simulink model "modelo_completo_2"  (R2023b)
settings: Solver=VariableStepAuto  StartTime=0.0  StopTime=300  MaxStep=5e-3  RelTol=1e-3
values from neighbouring files (symbols this model uses):
  P_p = 3    [constantes.m]
libraries: simulink x3
settings Model: Creator=Nahuel  LastModifiedBy=Nahuel

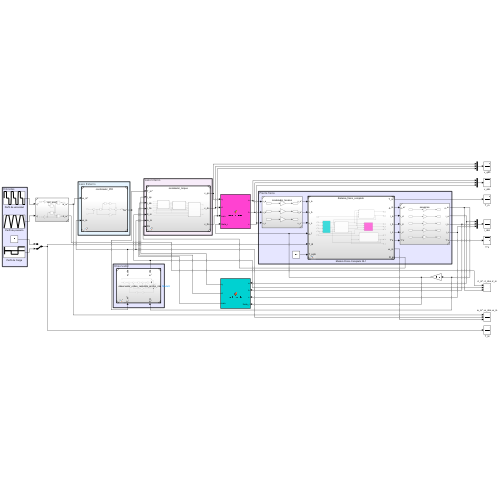
[thumbnail: Simulink's stored preview of the top-level diagram]
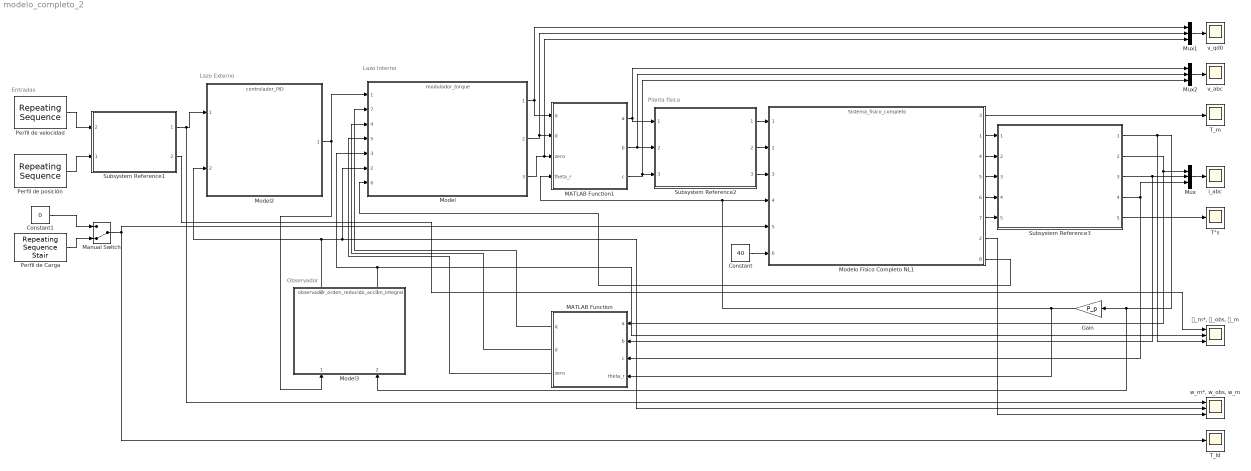
== system modelo_completo_2 ==
  note: Entradas
  note: Observador
  note: Lazo Externo
  note: Lazo Interno
  note: Planta física
  Constant : Constant  Value=40
  Constant1 : Constant  Value=0
  Gain : Gain  Gain=P_p
  MATLAB Function : MATLAB Function  TreatAsAtomicUnit=on
  MATLAB Function1 : MATLAB Function  TreatAsAtomicUnit=on
  Manual Switch : ManualSwitch  CurrentSetting=0
  Model : ModelReference  ModelNameDialog=modulador_torque.slx  SimulationMode=Normal  ModelReferenceVersion=1.5
      settings: PortSchema="{\"entries\":[{\"content\":{\"sides\":[{\"content\":{\"connectorIds\":[\"In1\",\"In7\",\"In4\",\"In5\",\"In3\",\"In2\",\"In6\"]},\"type\":\"ConnectorPlacement.EquallySpacedRectSide\",\"uuid\":\"1a431848-1219-464b-b81f-d5d4488f04a3\"},{\"content\":{\"connectorIds\":[\"Out1\",\"Out2\",\"Out3\"],\"side\":\"RIGHT\"},\"type\":\"ConnectorPlacement.EquallySpacedRectSide\",\"uuid\":\"e053d15c-f22a-49f8-bced-b1d540005571\"},{\"content\":{\"side\":\"TOP\"},\"type\":\"ConnectorPlacement.EquallySpacedRectSide\",\"uuid\":\"c0bb0860-826d-4b96-be85-5f71270b24f4\"}]},\"type\":\"ConnectorPlacement.EquallySpacedConnector\",\"uuid\":\"58d9e38e-69db-499f-b916-cb0043d9bf4b\"}],\"packageUris\":[\"http://schema.mathworks.com/mf0/Connector/R2020b\"],\"version\":\"1.0\"}"
  Model2 : ModelReference  ModelNameDialog=controlador_PID.slx  SimulationMode=Normal  ModelReferenceVersion=1.1
  Model3 : ModelReference  ModelNameDialog=observador_orden_reducido_accion_integral.slx  SimulationMode=Normal  ModelReferenceVersion=1.1
      settings: PortSchema="{\"entries\":[{\"content\":{\"sides\":[{\"content\":{\"connectorIds\":[\"In1\",\"In2\"]},\"type\":\"ConnectorPlacement.EquallySpacedRectSide\",\"uuid\":\"c19d64db-c009-4e99-a567-a0914790954a\"},{\"content\":{\"connectorIds\":[\"Out2\",\"Out1\"],\"side\":\"RIGHT\"},\"type\":\"ConnectorPlacement.EquallySpacedRectSide\",\"uuid\":\"cbca13ad-6906-458f-be0e-e9985fc9efad\"},{\"content\":{\"side\":\"TOP\"},\"type\":\"ConnectorPlacement.EquallySpacedRectSide\",\"uuid\":\"80bfb594-e700-4e7e-a208-88d990a8c4c7\"}]},\"type\":\"ConnectorPlacement.EquallySpacedConnector\",\"uuid\":\"c823fcd9-73b6-46d5-8b48-d21dc5db47ca\"}],\"packageUris\":[\"http://schema.mathworks.com/mf0/Connector/R2020b\"],\"version\":\"1.0\"}"
  Modelo Físico Completo NL1 : ModelReference  ModelNameDialog=Sistema_fisico_completo.slx  SimulationMode=Normal  ModelReferenceVersion=1.18
      settings: PortSchema="{\"entries\":[{\"content\":{\"sides\":[{\"content\":{\"connectorIds\":[\"In1\",\"In2\",\"In3\",\"In4\",\"In5\",\"In6\"]},\"type\":\"ConnectorPlacement.EquallySpacedRectSide\",\"uuid\":\"c38844a2-9b74-4da6-b9ce-d4868a84fb83\"},{\"content\":{\"connectorIds\":[\"Out3\",\"Out1\",\"Out4\",\"Out5\",\"Out6\",\"Out7\",\"Out2\",\"Out8\"],\"side\":\"RIGHT\"},\"type\":\"ConnectorPlacement.EquallySpacedRectSide\",\"uuid\":\"32cfc208-0644-4e1b-b9a9-83e6ff95cf9d\"},{\"content\":{\"side\":\"TOP\"},\"type\":\"ConnectorPlacement.EquallySpacedRectSide\",\"uuid\":\"4d8c9d59-309f-4ead-ae08-3f9c9c92e1b5\"}]},\"type\":\"ConnectorPlacement.EquallySpacedConnector\",\"uuid\":\"12663ecb-c0ca-4a2a-9423-b019766269d5\"}],\"packageUris\":[\"http://schema.mathworks.com/mf0/Connector/R2020b\"],\"version\":\"1.0\"}"
  Mux : Mux  Inputs=3
  Mux1 : Mux  Inputs=3
  Mux2 : Mux  Inputs=3
  Perfil de Carga : simulink/Sources/Repeating Sequence Stair  OutValues=[0 -5 5].'  tsamp=5  OutMin=[]  OutMax=[]  OutDataTypeStr=double  OutputDataTypeScalingMode=double  OutDataType=fixdt(0,8)  ConRadixGroup=Best Precision: Vector-wise  OutScaling=2^-12
  Perfil de posición : simulink/Sources/Repeating Sequence  rep_seq_t=[0 5 10 15]  rep_seq_y=[0 2*pi 2*pi 0]
  Perfil de velocidad : simulink/Sources/Repeating Sequence  rep_seq_t=[0 0.1 4.9 5 10 10.1 14.9 15]  rep_seq_y=[0 1.2566 1.2566 0 0 -1.2566 -1.2566 0]
  Subsystem Reference1 : Subsystem  ReferencedSubsystem=set_point
      settings: PortSchema="{\"entries\":[{\"content\":{\"sides\":[{\"content\":{\"connectorIds\":[\"In2\",\"In1\"]},\"type\":\"ConnectorPlacement.EquallySpacedRectSide\",\"uuid\":\"88e11a35-b720-4f74-932b-4aeb2d5e00b8\"},{\"content\":{\"connectorIds\":[\"Out1\",\"Out2\"],\"side\":\"RIGHT\"},\"type\":\"ConnectorPlacement.EquallySpacedRectSide\",\"uuid\":\"e8de25d9-7d20-45a0-a221-6f807a46a39c\"},{\"content\":{\"side\":\"TOP\"},\"type\":\"ConnectorPlacement.EquallySpacedRectSide\",\"uuid\":\"c3c686d5-d3fa-4802-9f1b-650cab118ebd\"}]},\"type\":\"ConnectorPlacement.EquallySpacedConnector\",\"uuid\":\"961bc988-ee92-4957-9464-cf01ec4baf2c\"}],\"packageUris\":[\"http://schema.mathworks.com/mf0/Connector/R2020b\"],\"version\":\"1.0\"}"
  Subsystem Reference2 : Subsystem  ReferencedSubsystem=modulador_tension
  Subsystem Reference3 : Subsystem  ReferencedSubsystem=sensores
  T_ld : Scope
  T_m : Scope
  T°s : Scope
  i_abc : Scope
  v_abc : Scope
  v_qd0 : Scope
  "w_m*, w_obs, w_m" : Scope  NumInputPorts=3
  "𝜃_m*, 𝜃_obs, 𝜃_m" : Scope  NumInputPorts=3
  wires:
  Subsystem Reference2/1 -> Modelo Físico Completo NL1/1
  Subsystem Reference2/2 -> Modelo Físico Completo NL1/2
  Subsystem Reference2/3 -> Modelo Físico Completo NL1/3
  Modelo Físico Completo NL1/1 -> Subsystem Reference3/1
  Modelo Físico Completo NL1/4 -> Subsystem Reference3/2
  Modelo Físico Completo NL1/5 -> Subsystem Reference3/3
  Modelo Físico Completo NL1/6 -> Subsystem Reference3/4
  Modelo Físico Completo NL1/7 -> Subsystem Reference3/5
  Subsystem Reference3/1 -> Model3/2, Gain/1, "𝜃_m*, 𝜃_obs, 𝜃_m"/3
  Gain/1 -> Modelo Físico Completo NL1/4, MATLAB Function1/4(theta_r), MATLAB Function/4(theta_r)
  Model2/1 -> Model3/1, Model/1
  Model3/1 -> Model/3, "𝜃_m*, 𝜃_obs, 𝜃_m"/2
  Model3/2 -> Model/2, "w_m*, w_obs, w_m"/2, Model2/2
  Subsystem Reference3/2 -> MATLAB Function/1(a), Mux/1
  Subsystem Reference3/3 -> MATLAB Function/2(b), Mux/2
  Subsystem Reference3/4 -> MATLAB Function/3(c), Mux/3
  Mux/1 -> i_abc/1
  Modelo Físico Completo NL1/3 -> T_m/1
  Subsystem Reference3/5 -> T°s/1
  MATLAB Function/1(q) -> Model/7
  MATLAB Function/2(d) -> Model/4
  MATLAB Function/3(zero) -> Model/5
  Constant/1 -> Modelo Físico Completo NL1/6
  Model/2 -> Mux1/2, MATLAB Function1/2(d)
  Mux2/1 -> v_abc/1
  Model/3 -> MATLAB Function1/3(zero), Mux1/3
  Model/1 -> MATLAB Function1/1(q), Mux1/1
  Mux1/1 -> v_qd0/1
  MATLAB Function1/3(c) -> Mux2/3, Subsystem Reference2/3
  MATLAB Function1/2(b) -> Subsystem Reference2/2, Mux2/2
  MATLAB Function1/1(a) -> Subsystem Reference2/1, Mux2/1
  Subsystem Reference1/2 -> "𝜃_m*, 𝜃_obs, 𝜃_m"/1
  Modelo Físico Completo NL1/8 -> Model/6
  Subsystem Reference1/1 -> Model2/1, "w_m*, w_obs, w_m"/1
  Modelo Físico Completo NL1/2 -> "w_m*, w_obs, w_m"/3
  Constant1/1 -> Manual Switch/1
  Perfil de Carga/1 -> Manual Switch/2
  Manual Switch/1 -> T_ld/1, Modelo Físico Completo NL1/5
  Perfil de posición/1 -> Subsystem Reference1/1
  Perfil de velocidad/1 -> Subsystem Reference1/2

== matlab function modelo_completo_2/MATLAB Function1 ==
  data: q input; a output; d input; zero input; theta_r input; b output; c output
function [a, b, c] = park_inversa(q, d, zero, theta_r)
    % Transformación de Park Inversa
    % Entradas:
    %   d, q, z: Coordenadas en el marco rotatorio
    %   theta: Ángulo en radianes
    % Salidas:
    %   a, b, c: Valores trifásicos reconstruidos
    
    % Constantes
    alpha = 2 * pi / 3; % Desplazamiento angular entre fases
    
    % Cálculo de valores trifásicos
    a = q * cos(theta_r) + d * sin(theta_r) + zero;
    b = q * cos(theta_r - alpha) + d * sin(theta_r - alpha) + zero;
    c = q * cos(theta_r + alpha) + d * sin(theta_r + alpha) + zero;
end

== matlab function modelo_completo_2/MATLAB Function ==
  data: q output; a input; d output; b input; c input; theta_r input; zero output
function [q, d, zero] = park_directa(a, b, c, theta_r)
    % Transformación de Park Directa
    % Entradas:
    %   a, b, c: Valores trifásicos
    %   theta: Ángulo en radianes
    % Salidas:
    %   d, q, z: Coordenadas en el marco rotatorio
    
    % Constantes
    alpha = 2 * pi / 3; % Desplazamiento angular entre fases
    k = 2 / 3; % Escala para invarianza
    
    % Cálculo de coordenadas d, q, z
    q = k * (a * cos(theta_r) + b * cos(theta_r - alpha) + c * cos(theta_r + alpha));
    d = k * (a * sin(theta_r) + b * sin(theta_r - alpha) + c * sin(theta_r + alpha));
    zero = k * (a * 1/2 + b * 1/2 + c * 1/2);
end
